simulink model "hw3nonlinearcontrolsim"  (R2025b)
settings: Solver=VariableStepAuto  StartTime=0.0  StopTime=10  RelTol=1e-3
libraries: roblocks x1
settings Model: Creator=ckitt  LastModifiedBy=Jaxba

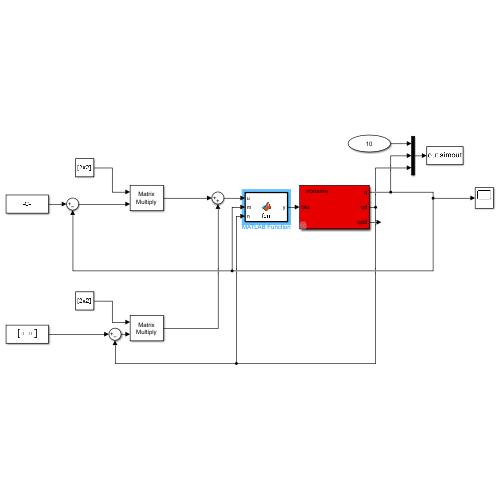
[thumbnail: Simulink's stored preview of the top-level diagram]
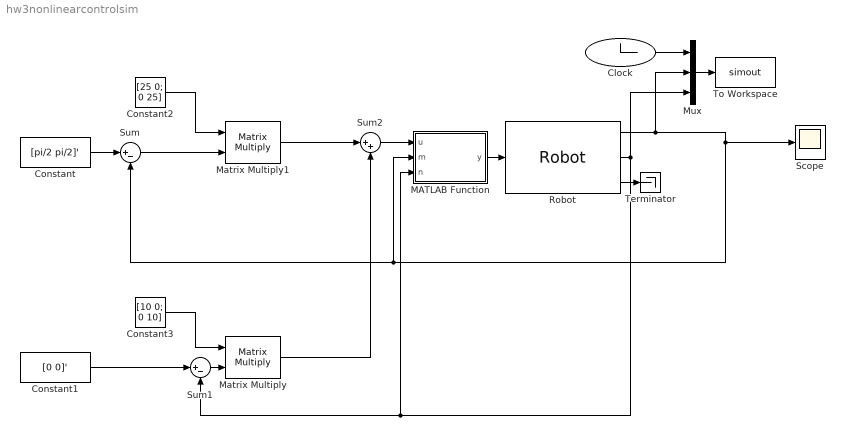
== system hw3nonlinearcontrolsim ==
  Clock : Clock
  Constant : Constant  Value=[pi/2 pi/2]'
  Constant1 : Constant  Value=[0 0]'
  Constant2 : Constant  Value=[25 0; 0 25]
  Constant3 : Constant  Value=[10 0; 0 10]
  MATLAB Function : MATLAB Function  TreatAsAtomicUnit=on
  Matrix Multiply : Product  Multiplication=Matrix(*)
  Matrix Multiply1 : Product  Multiplication=Matrix(*)
  Mux : Mux  Inputs=3
  Robot : roblocks/Robot  robot=SCURRbot  q0=[0 0]
  Scope : Scope
      settings: ActiveDisplayYMinimum=-0.16509461069838527  ActiveDisplayYMaximum=1.9298843670094636
  Sum : Sum  Inputs=|+-
  Sum1 : Sum  Inputs=|+-
  Sum2 : Sum  Inputs=|++
  Terminator : Terminator
  To Workspace : ToWorkspace  VariableName=simout  SampleTime=-1
  wires:
  Robot/3 -> Terminator/1
  Clock/1 -> Mux/1
  Mux/1 -> To Workspace/1
  Robot/1 -> Mux/2, Scope/1, MATLAB Function/2(m), Sum/2
  Constant/1 -> Sum/1
  Constant1/1 -> Sum1/1
  Robot/2 -> Mux/3, MATLAB Function/3(n), Sum1/2
  Sum1/1 -> Matrix Multiply/2
  Constant3/1 -> Matrix Multiply/1
  Sum/1 -> Matrix Multiply1/2
  Constant2/1 -> Matrix Multiply1/1
  Matrix Multiply1/1 -> Sum2/1
  Matrix Multiply/1 -> Sum2/2
  Sum2/1 -> MATLAB Function/1(u)
  MATLAB Function/1(y) -> Robot/1

== matlab function hw3nonlinearcontrolsim/MATLAB Function ==
  data: u input; y output; m input; n input
function y = fcn(u, m, n)

L1 = 1; L2 = 1;
m1 = 3; m2 = 3; B1 = 3; B2 = 3;


m11 = m2+2*m2*cos(m(2))+(m1+m2);
m12 = m2+m2*cos(m(2));
m21 = m2+m2*cos(m(2));
m22 = m2;
M = [m11 m12; m21 m22];

%V1 = -m2*sin(m(2))*n(2);
%V2 = m2*sin(m(2))*n(1);

V1 = -0.5*m1*sin(m(2))*n(2);
V2 = -0.5*sin(m(2))*(n(1)+n(2));
V = [V1; V2];

B = [B1*n(1); B2*n(2)];

y = M*u + V + B;
